simulink model "controller"  (R2021b)
settings: Solver=VariableStepAuto  StartTime=0.0  StopTime=10.0  RelTol=1e-3
settings Model: Creator=jcron  LastModifiedBy=jcron

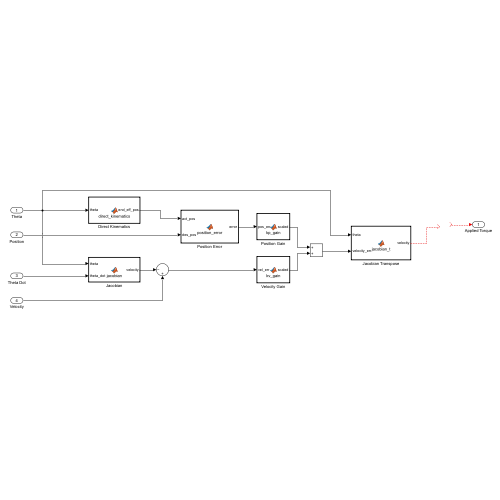
[thumbnail: Simulink's stored preview of the top-level diagram]
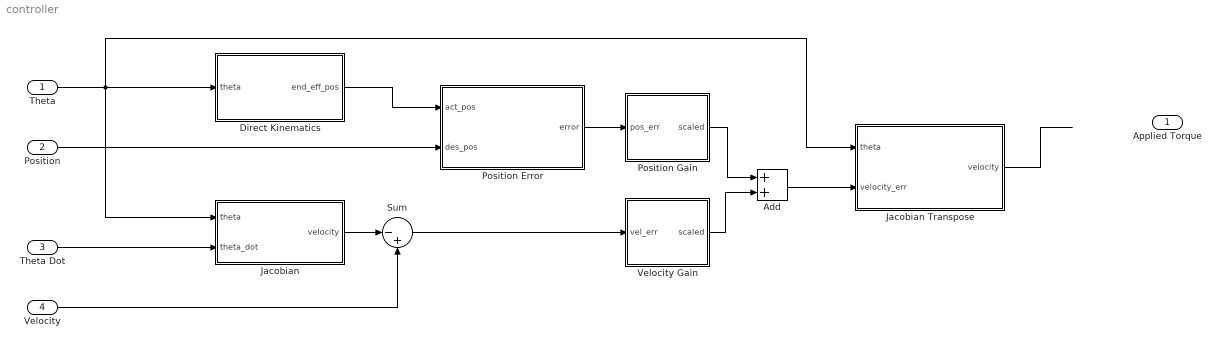
== system controller ==
  Theta : Inport  PortDimensions=DOF
  Position : Inport  Port=2
  Theta Dot : Inport  Port=3  PortDimensions=DOF
  Velocity : Inport  Port=4  PortDimensions=[6 1]
  Add : Sum
  Direct Kinematics : MATLAB Function  TreatAsAtomicUnit=on
  Jacobian : MATLAB Function  TreatAsAtomicUnit=on
  Jacobian Transpose : MATLAB Function  TreatAsAtomicUnit=on
  Position Error : MATLAB Function  TreatAsAtomicUnit=on
  Position Gain : MATLAB Function  TreatAsAtomicUnit=on
  Sum : Sum  Inputs=|-+
  Velocity Gain : MATLAB Function  TreatAsAtomicUnit=on
  Applied Torque : Outport
  wires:
  Direct Kinematics/1(end_eff_pos) -> Position Error/1(act_pos)
  Position/1 -> Position Error/2(des_pos)
  Theta/1 -> Jacobian Transpose/1(theta), Direct Kinematics/1(theta), Jacobian/1(theta)
  Jacobian Transpose/1(velocity) -> ?
  Theta Dot/1 -> Jacobian/2(theta_dot)
  Velocity Gain/1(scaled) -> Add/2
  Add/1 -> Jacobian Transpose/2(velocity_err)
  ? -> Applied Torque/1
  Jacobian/1(velocity) -> Sum/1
  Velocity/1 -> Sum/2
  Position Gain/1(scaled) -> Add/1
  Position Error/1(error) -> Position Gain/1(pos_err)
  Sum/1 -> Velocity Gain/1(vel_err)

== matlab function controller/Direct Kinematics ==
  data: theta input size=[3 1]; end_eff_pos output
function end_eff_pos = direct_kinematics(theta)
end_eff_pos = zeros(4, 4);
[end_eff_frame, end_eff_origin] = directKinematics(theta);
end_eff_pos = [
    end_eff_frame end_eff_origin;
    zeros(1, 3) 1
];

== matlab function controller/Position Error ==
  data: act_pos input size=[4 4]; des_pos input size=[4 4]; error output
function error  = position_error(act_pos, des_pos)
error = zeros(6, 1);
desired_frame = des_pos(1:3, 1:3);
desired_origin = des_pos(1:3, 4);

actual_frame = act_pos(1:3, 1:3);
actual_origin = act_pos(1:3, 4);

trans_err = desired_origin - actual_origin;
rotational_error = rotm2axang(desired_frame' * actual_frame);

rot_err = rotational_error(1:3)';
rot_err = rotational_error(4) .* rot_err;

error = [trans_err; rot_err];

== matlab function controller/Jacobian ==
  data: theta input; velocity output; theta_dot input
function velocity = jacobian(theta, theta_dot)
velocity = zeros(6, 1);
J = jacobian(theta);
velocity = J * theta_dot;

== matlab function controller/Jacobian Transpose ==
  data: theta input; velocity output; velocity_err input
function velocity = jacobian_t(theta, velocity_err)
velocity = zeros(3, 1);
J = jacobian(theta);
velocity = J' * velocity_err;

== matlab function controller/Position Gain ==
  data: pos_err input size=[6 1]; scaled output; Kp parameter
function scaled = kp_gain(pos_err, Kp)
scaled = zeros(6, 1);
scaled = Kp * pos_err;

== matlab function controller/Velocity Gain ==
  data: vel_err input size=[6 1]; scaled output; Kv parameter
function scaled = kv_gain(vel_err, Kv)
scaled = zeros(6, 1);
scaled = Kv * vel_err;
